simulink model "beluga_yaw_model"  (R2016b)
settings: Solver=ode45  StartTime=0.0  StopTime=5  RelTol=1e-8  AbsTol=1e-10
values from neighbouring files (symbols this model uses):
  A = v_lin(ind)-slope*t_step(ind)    [calculate_PID.m]    (also in spline_vel.m = [   to^3,   to^2,   to, 1; spline_yaw.m = [   to^5,   to^4,  to^3,   to^2,   to, 1)
  Kd = double(real(Kd.Kd))    [phasePD.m]    (also in run_yaw.m = 3.47)
  Kp = 1.2/A    [calculate_PID.m]    (also in phasePD.m = double(real(Kp)); run_yaw.m = 2.17)
  td = 0.11    [phasePD.m]
undefined symbols (not defined in the file or in its folder): Ki, tau
settings Model: Creator=bright  LastModifiedBy=bright
settings DataIOCC: SaveFormat=Array  SignalLoggingSaveFormat=ModelDataLogs  Refine=10
settings OptimizationCC: BlockReduction=off  BooleanDataType=off
settings DebuggingCC: SaveWithParameterizedLinksMsg=none  UnderspecifiedInitializationDetection=Classic  MergeDetectMultiDrivingBlocksExec=none  SignalResolutionControl=TryResolveAllWithWarning  MultiTaskDSMMsg=warning  MultiTaskCondExecSysMsg=none
settings HardwareCC: TargetUnknown=on
settings ModelReferenceCC: PropagateSignalLabelsOutOfModel=off
settings GRTTargetCC: TargetLangStandard=C89/C90 (ANSI)  CombineOutputUpdateFcns=off  GRTInterface=on

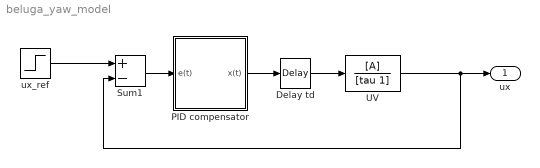
== system beluga_yaw_model ==
  Delay td : TransportDelay  DelayTime=td
  PID compensator : Subsystem
  Sum1 : Sum  Inputs=+-  SaturateOnIntegerOverflow=on  InputSameDT=on  OutDataTypeStr=Inherit: Same as first input
  UV : TransferFcn  Numerator=[A]  Denominator=[tau 1]
  ux_ref : Step  Time=0  After=0.5
  ux : Outport
  wires:
  Delay td/1 -> UV/1
  ux_ref/1 -> Sum1/1
  UV/1 -> ux/1, Sum1/2
  Sum1/1 -> PID compensator/1(e(t))
  PID compensator/1(x(t)) -> Delay td/1

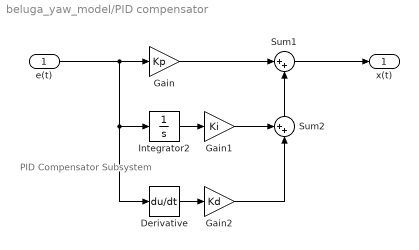
== system beluga_yaw_model/PID compensator ==
  note: PID Compensator
      | Subsystem
  e(t) : Inport
  Derivative : Derivative
  Gain : Gain  Gain=Kp
  Gain1 : Gain  Gain=Ki
  Gain2 : Gain  Gain=Kd
  Integrator2 : Integrator
  Sum1 : Sum  Inputs=|++
  Sum2 : Sum  Inputs=++|
  x(t) : Outport
  wires:
  Integrator2/1 -> Gain1/1
  Gain1/1 -> Sum2/1
  Sum2/1 -> Sum1/2
  Gain/1 -> Sum1/1
  Sum1/1 -> x(t)/1
  Gain2/1 -> Sum2/2
  e(t)/1 -> Gain/1, Integrator2/1, Derivative/1
  Derivative/1 -> Gain2/1
